simulink model "smcSL"  (R2020b)
settings: Solver=VariableStepAuto  StartTime=0.0  StopTime=10
undefined symbols (not defined in the file): a, beta, d1, d2, delta, DZ, I, km, MAX_PWM, miu, wb, wcp, wm
settings Model: Creator=andre  LastModifiedBy=andre
settings SolverCC: ZeroCrossAlgorithm=Adaptive
settings DebuggingCC: IgnoredZcDiagnostic=none

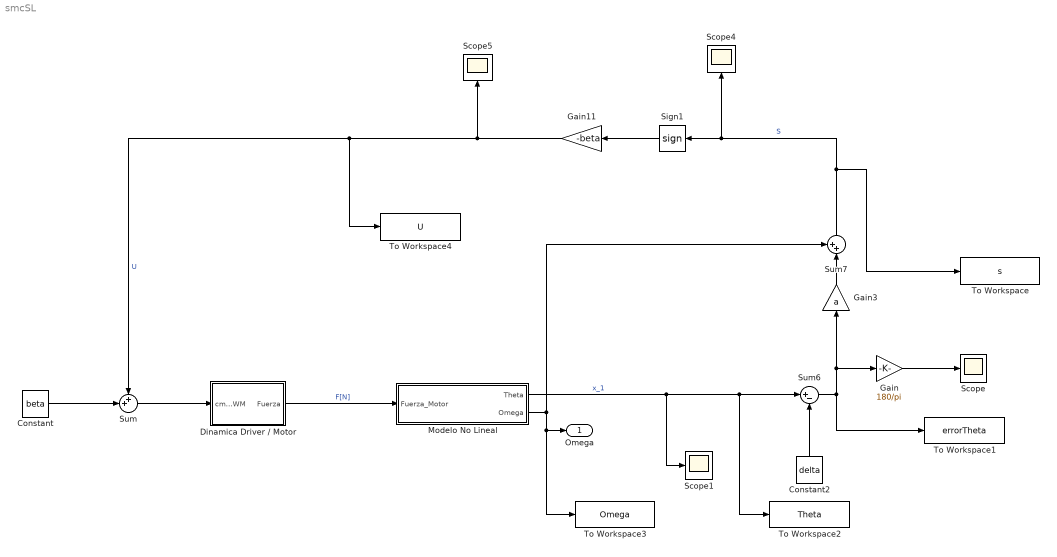
== system smcSL ==
  Constant : Constant  Value=beta
  Constant2 : Constant  Value=delta
  Dinamica Driver / Motor : Subsystem
  Gain : Gain  Gain=180/pi
  Gain11 : Gain  Gain=-beta
  Gain3 : Gain  Gain=a
  Modelo No Lineal : Subsystem
  Scope{,1,4..5} (4 alike) : Scope
  Sign1 : Signum  ZeroCross=off
  Sum : Sum  Inputs=++|
  Sum6 : Sum  Inputs=|+-
  Sum7 : Sum  Inputs=++|
  To Workspace : ToWorkspace  VariableName=s  SaveFormat=Timeseries  SampleTime=-1
  To Workspace1 : ToWorkspace  VariableName=errorTheta  SaveFormat=Timeseries  SampleTime=-1
  To Workspace2 : ToWorkspace  VariableName=Theta  SaveFormat=Timeseries  SampleTime=-1
  To Workspace3 : ToWorkspace  VariableName=Omega  SaveFormat=Timeseries  SampleTime=-1
  To Workspace4 : ToWorkspace  VariableName=U  SaveFormat=Timeseries  SampleTime=-1
  Omega : Outport
  wires:
  Sign1/1 -> Gain11/1
  Gain3/1 -> Sum7/2
  Sum6/1 -> Gain/1, Gain3/1, To Workspace1/1
  Modelo No Lineal/1(Theta) -> Scope1/1, To Workspace2/1, Sum6/1  "x_1"
  Sum7/1 -> To Workspace/1, Scope4/1, Sign1/1  "S"
  Gain11/1 -> To Workspace4/1, Sum/1, Scope5/1  "U"
  Constant2/1 -> Sum6/2
  Dinamica Driver / Motor/1(Fuerza) -> Modelo No Lineal/1(Fuerza_Motor)  "F[N]"
  Modelo No Lineal/2(Omega) -> Sum7/1, To Workspace3/1, Omega/1
  Constant/1 -> Sum/2
  Sum/1 -> Dinamica Driver / Motor/1(cmd_PWM)
  Gain/1 -> Scope/1

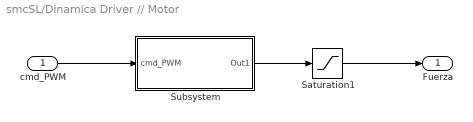
== system smcSL/Dinamica Driver // Motor ==
  cmd_PWM : Inport
  Saturation1 : Saturate  UpperLimit=MAX_PWM  ZeroCross=off
  Subsystem : Subsystem
  Fuerza : Outport
  wires:
  Saturation1/1 -> Fuerza/1
  cmd_PWM/1 -> Subsystem/1(cmd_PWM)
  Subsystem/1(Out1) -> Saturation1/1

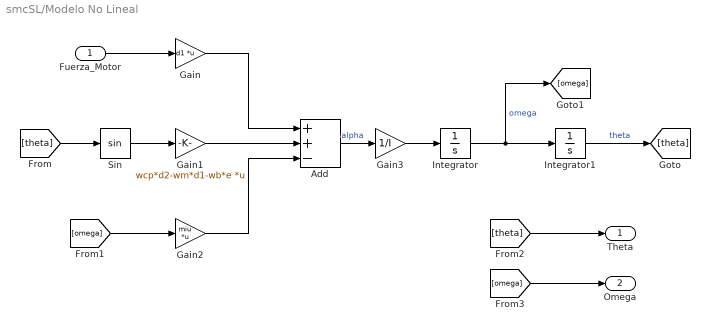
== system smcSL/Modelo No Lineal ==
  Fuerza_Motor : Inport
  Add : Sum  Inputs=++-
  Gain : Gain  Gain=d1  Multiplication=Matrix(K*u)
  Gain1 : Gain  Gain=wcp*d2-wm*d1-wb*e  Multiplication=Matrix(K*u)
  Gain2 : Gain  Gain=miu  Multiplication=Matrix(K*u)
  Gain3 : Gain  Gain=1/I
  Integrator : Integrator  ZeroCross=off
  Integrator1 : Integrator  InitialCondition=pi/2  ZeroCross=off
  Sin : Trigonometry  ApproximationMethod=CORDIC
  Theta : Outport
  Omega : Outport  Port=2
  wires:
  [omega] -> Omega/1
  Gain1/1 -> Add/2
  Integrator/1 -> [omega], Integrator1/1  "omega"
  Fuerza_Motor/1 -> Gain/1
  Integrator1/1 -> [theta]  "theta"
  Gain2/1 -> Add/3
  Gain/1 -> Add/1
  Add/1 -> Gain3/1  "alpha"
  [theta] -> Sin/1
  [omega] -> Gain2/1
  [theta] -> Theta/1
  Sin/1 -> Gain1/1
  Gain3/1 -> Integrator/1

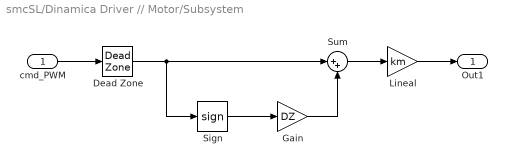
== system smcSL/Dinamica Driver // Motor/Subsystem ==
  cmd_PWM : Inport
  Dead Zone : DeadZone  LowerValue=-DZ  UpperValue=DZ  ZeroCross=off  SaturateOnIntegerOverflow=on
  Gain : Gain  Gain=DZ
  Lineal : Gain  Gain=km
  Sign : Signum  ZeroCross=off
  Sum : Sum  Inputs=|++
  Out1 : Outport
  wires:
  cmd_PWM/1 -> Dead Zone/1
  Dead Zone/1 -> Sum/1, Sign/1
  Sum/1 -> Lineal/1
  Sign/1 -> Gain/1
  Gain/1 -> Sum/2
  Lineal/1 -> Out1/1
